simulink subsystem "DCServoMotor_SubSystem"  (R2020b)
settings: Solver=VariableStepAuto  StartTime=0.0  StopTime=10.0  RelTol=1e-3
undefined symbols (not defined in the file or in its folder): sens
settings Model: Creator=umberto  LastModifiedBy=umberto

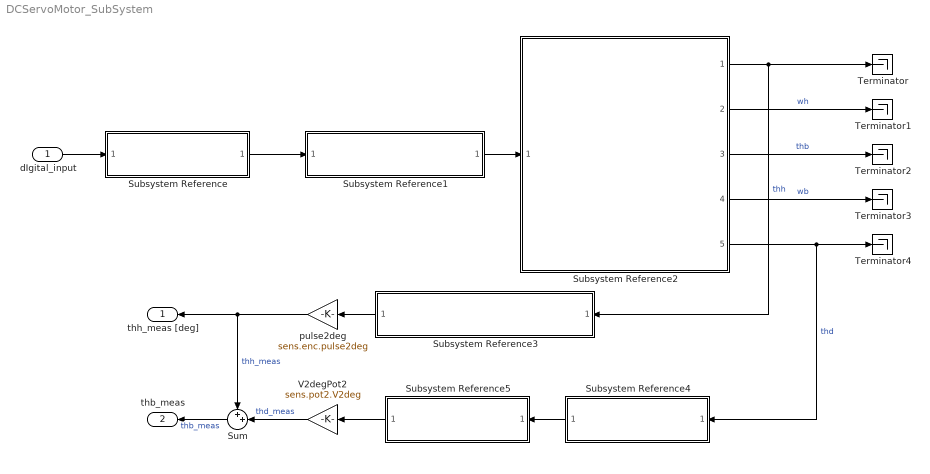
== system DCServoMotor_SubSystem ==
  dIgital_input : Inport
  Subsystem Reference : Subsystem  ReferencedSubsystem=DAC_SubSystem
  Subsystem Reference1 : Subsystem  ReferencedSubsystem=Driver_SubSystem
  Subsystem Reference2 : Subsystem  ReferencedSubsystem=DCGearmotorResonant_SubSystem
  Subsystem Reference3 : Subsystem  ReferencedSubsystem=Encoder_SubSystem
  Subsystem Reference4 : Subsystem  ReferencedSubsystem=Potentiometer2_SubSystem
  Subsystem Reference5 : Subsystem  ReferencedSubsystem=ADC_SubSystem
  Sum : Sum  Inputs=++|
  Terminator{,1..4} (5 alike) : Terminator
  V2degPot2 : Gain  Gain=sens.pot2.V2deg
  pulse2deg : Gain  Gain=sens.enc.pulse2deg
  thh_meas [deg] : Outport
  thb_meas : Outport  Port=2
  wires:
  dIgital_input/1 -> Subsystem Reference/1
  Subsystem Reference1/1 -> Subsystem Reference2/1
  Subsystem Reference2/2 -> Terminator1/1  "wh"
  Subsystem Reference3/1 -> pulse2deg/1
  pulse2deg/1 -> Sum/1, thh_meas [deg]/1  "thh_meas"
  Subsystem Reference/1 -> Subsystem Reference1/1
  Sum/1 -> thb_meas/1  "thb_meas"
  V2degPot2/1 -> Sum/2  "thd_meas"
  Subsystem Reference5/1 -> V2degPot2/1
  Subsystem Reference4/1 -> Subsystem Reference5/1
  Subsystem Reference2/1 -> Subsystem Reference3/1, Terminator/1  "thh"
  Subsystem Reference2/5 -> Subsystem Reference4/1, Terminator4/1  "thd"
  Subsystem Reference2/4 -> Terminator3/1  "wb"
  Subsystem Reference2/3 -> Terminator2/1  "thb"
